simulink model "Topic6_SwitchLed"  (R2021a)
settings: Solver=FixedStepDiscrete  StartTime=0.0  StopTime=inf  FixedStep=0.5  RelTol=1e-3  EnableMultiTasking=on
settings Model: SILPILModeSetting=veronly  ExtModeTrigDuration=2  Creator=Michael_Ibrahim  LastModifiedBy=Michael_Ibrahim
settings DataIOCC: ReturnWorkspaceOutputs=off
settings OptimizationCC: EnableMemcpy=off  LifeSpan=1  MaxStackSize=64  EfficientTunableParamExpr=on
settings DebuggingCC: UnderspecifiedInitializationDetection=Classic  MergeDetectMultiDrivingBlocksExec=none  SFMachineParentedDataDiag=warning  ArithmeticOperatorsInVariantConditions=warning
settings HardwareCC: ProdBitPerInt=16  ProdBitPerPointer=16  ProdBitPerSizeT=16  ProdBitPerPtrDiffT=16  ProdLargestAtomicFloat=None  ProdWordSize=8  ProdHWDeviceType=Atmel->AVR
settings ModelReferenceCC: PropagateSignalLabelsOutOfModel=off
settings SFSimCC: MATLABDynamicMemAlloc=off  CustomCodeUndefinedFunction=UseInterfaceOnly
settings RTWCC: SystemTargetFile=ert.tlc  HardwareBoard=Arduino Uno  GenCodeOnly=on  TemplateMakefile=ert_default_tmf  GenerateReport=on  Toolchain=Arduino AVR  IncludeHyperlinkInReport=on  LaunchReport=on  GenerateTraceInfo=on  GenerateTraceReport=on  GenerateTraceReportSl=on  GenerateTraceReportSf=on  GenerateTraceReportEml=on
settings CodeAppCC: ForceParamTrailComments=on  IgnoreCustomStorageClasses=off  OperatorAnnotations=on  SimulinkDataObjDesc=on  SFDataObjDesc=on  MATLABFcnDesc=on  InsertBlockDesc=on  StateflowObjectComments=on  MATLABSourceComments=on
settings ERTTargetCC: MultiwordLength=2048  SupportContinuousTime=on  SupportVariableSizeSignals=on  ExtModeStaticAllocSize=250

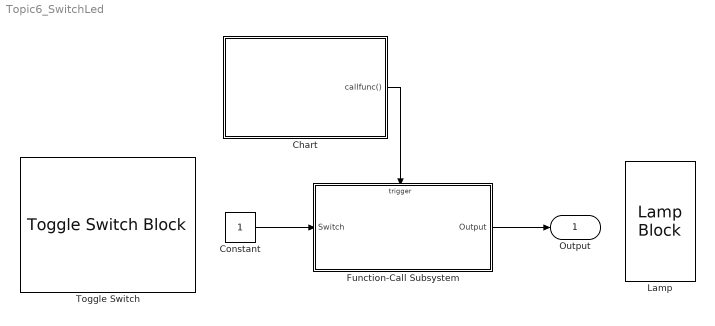
== system Topic6_SwitchLed ==
  Chart : Stateflow chart  TreatAsAtomicUnit=on
  Constant : Constant
  Function-Call Subsystem : Subsystem  TreatAsAtomicUnit=on
  Lamp : LampBlock
  Toggle Switch : ToggleSwitchBlock
      settings: Values={{'Off', 'On'}, [0 1]}
  Output : Outport
  wires:
  Chart/1(callfunc()) -> Function-Call Subsystem/Trigger
  Constant/1 -> Function-Call Subsystem/1(Switch)
  Function-Call Subsystem/1(Output) -> Output/1

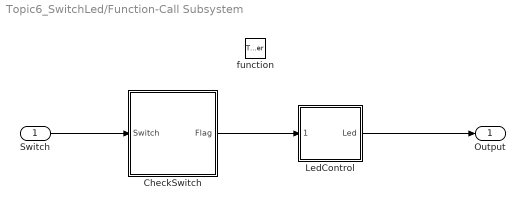
== system Topic6_SwitchLed/Function-Call Subsystem ==
  Switch : Inport
  function : TriggerPort  TriggerType=function-call  VariantControl=(inherit)
  CheckSwitch : Stateflow chart  TreatAsAtomicUnit=on
  LedControl : Stateflow chart  TreatAsAtomicUnit=on
  Output : Outport
  wires:
  Switch/1 -> CheckSwitch/1(Switch)
  CheckSwitch/1(Flag) -> LedControl/1(LedControl)
  LedControl/1(Led) -> Output/1

== stateflow chart Topic6_SwitchLed/Function-Call Subsystem/CheckSwitch ==
  (default) -> (junction 7) : % CheckButton
  (junction 7) -> (junction 8) [order 1] : [Switch == 1]
  (junction 7) -> (junction 9) [order 2] : {Flag = 0;}
  (junction 8) -> (junction 10) : {Flag = 1;}
  (junction 10) -> (junction 9)
  (junction 9) -> (junction 11)
  data: Switch input; Flag output

== stateflow chart Topic6_SwitchLed/Function-Call Subsystem/LedControl ==
  (default) -> (junction 7) : % LedControl
  (junction 7) -> (junction 8) [order 1] : [LedControl == 1]
  (junction 7) -> (junction 9) [order 2] : {Led = 0;}
  (junction 8) -> (junction 10) : {Led = 1;}
  (junction 10) -> (junction 9)
  (junction 9) -> (junction 11)
  data: LedControl input; Led output

== stateflow chart Topic6_SwitchLed/Chart ==
  state CallFunction
    en:
    du:
    ex:
  (default) -> CallFunction
  CallFunction -> CallFunction : [after(5,msec)]{callfunc;}
  events: callfunc output FUNCTION_CALL_EVENT
